simulink model "PM_fnc100_TestHarness_backup"  (R2022a)
settings: Solver=VariableStepAuto  StartTime=0.0  StopTime=10.0  RelTol=1e-3
values from neighbouring files (symbols this model uses):
  rate_ms = 10    [PM_fnc1000_tc01_iter01_testsignal_builder.m]    (also in PM_fnc21_tc01_iter01_testsignal_builder.m; PM_fnc22_tc01_iter01_testsignal_builder.m)
undefined symbols (not defined in the file or in its folder): cal_abs_ampslimit_hyst_A, cal_abs_ampslimit_thresh_A, cal_cell_heat2cool_factor, cal_Dchg_10sPL_expiry_dur_thresh_ms, cal_Dchg_50sPL_expiry_dur_thresh_ms, cal_Regen_10sPL_expiry_dur_thresh_ms, cal_Regen_50sPL_expiry_dur_thresh_ms, cal_table_cell_soc_percent, cal_table_cell_temp_degC
settings Model: Creator=306427  LastModifiedBy=306427

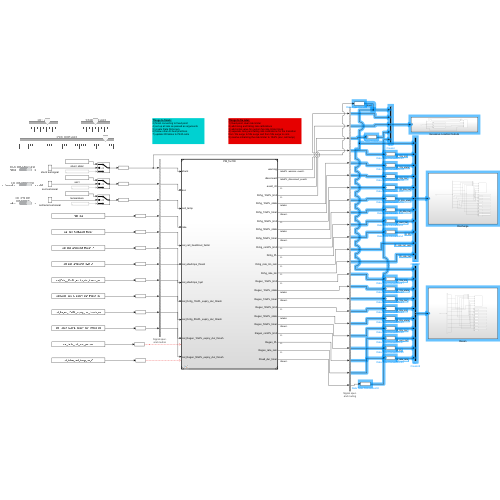
[thumbnail: Simulink's stored preview of the top-level diagram]
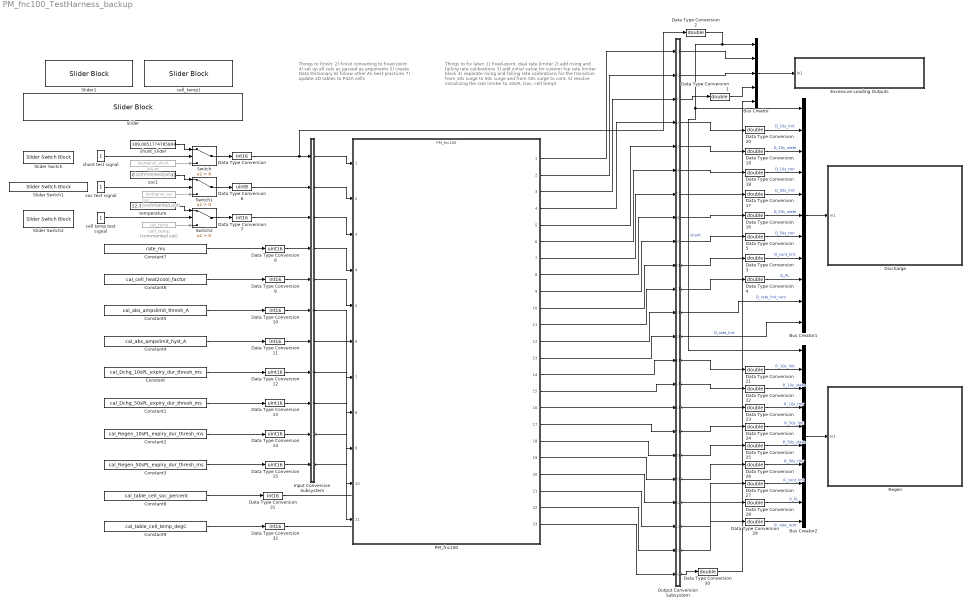
== system PM_fnc100_TestHarness_backup ==
  note: Things to finish:
      | 2) finish converting to fixed point
      | 4) set up all cals as passed as arguments
      | 5) create Data Dictionary
      | 6) follow other Ali best practices
      | 7) update 2D tables to P42A cells
  note: Things to fix later:
      | 1) fixed-point, dual rate limiter
      | 2) add rising and falling rate calibrations
      | 3) add initial value for custom fxp rate limiter block
      | 4) separate rising and falling rate calibrations for the transition from 10s surge to 50s surge and from 50s surge to cont.
      | 5) resolve initializing the rate limiter to 10sPL (soc, cell temp)
  Bus Creator : BusCreator  Inputs=5
  Bus Creator1 : BusCreator  Inputs=11
  Bus Creator2 : BusCreator  Inputs=10
  Constant : Constant  Value=cal_Dchg_10sPL_expiry_dur_thresh_ms
  Constant1 : Constant  Value=cal_Dchg_50sPL_expiry_dur_thresh_ms
  Constant2 : Constant  Value=cal_Regen_10sPL_expiry_dur_thresh_ms
  Constant3 : Constant  Value=cal_Regen_50sPL_expiry_dur_thresh_ms
  Constant4 : Constant  Value=cal_abs_ampslimit_hyst_A
  Constant5 : Constant  Value=cal_abs_ampslimit_thresh_A
  Constant6 : Constant  Value=cal_cell_heat2cool_factor
  Constant7 : Constant  Value=rate_ms
  Constant8 : Constant  Value=cal_table_cell_soc_percent
  Constant9 : Constant  Value=cal_table_cell_temp_degC
  Data Type Conversion{,7,9..11,31..32} (7 alike) : DataTypeConversion  OutDataTypeStr=int16  SaturateOnIntegerOverflow=off  RndMeth=Floor
  Data Type Conversion{1..5,16..30} (20 alike) : DataTypeConversion  OutDataTypeStr=double  SaturateOnIntegerOverflow=off  RndMeth=Floor
  Data Type Conversion{8,12..15} (5 alike) : DataTypeConversion  OutDataTypeStr=uint16  SaturateOnIntegerOverflow=off  RndMeth=Floor
  Data Type Conversion6 : DataTypeConversion  OutDataTypeStr=uint8  SaturateOnIntegerOverflow=off  RndMeth=Floor
  Discharge : Subsystem
  Excessive Loading Outputs : Subsystem
  Input Conversion Subsystem : Subsystem  Tag=__SLT_ICS__  Description=|
      | Signal spec.
      | and routing
      settings: AttributesFormatString=%<Description>
  Output Conversion Subsystem : Subsystem  Tag=__SLT_OCS__  Description=|
      | Signal spec.
      | and routing
      settings: AttributesFormatString=%<Description>
  PM_fnc100 : ModelReference  ModelNameDialog=PM_fnc100  SimulationMode=Normal  ModelReferenceVersion=1.79
  Regen : Subsystem
  Slider : SliderBlock  ScaleMin=-1700  ScaleMax=+500
  Slider Switch : SliderSwitchBlock
      settings: Values={{'from wksp', 'slider'}, [0 1]}
  Slider Switch1 : SliderSwitchBlock
      settings: Values={{'soc from wksp', 'soc slider'}, [0 1]}
  Slider Switch2 : SliderSwitchBlock
      settings: Values={{'from wksp', 'slider'}, [0 1]}
  Slider1 : SliderBlock
  Switch : Switch  Criteria=u2 > Threshold  SaturateOnIntegerOverflow=off  InputSameDT=off
  Switch1 : Switch  Criteria=u2 > Threshold  SaturateOnIntegerOverflow=off  InputSameDT=off
  Switch2 : Switch  Criteria=u2 > Threshold  SaturateOnIntegerOverflow=off  InputSameDT=off
  cell temp test signal : Constant
  cell_temp : FromWorkspace  Commented=on  VariableName=cell_temp  OutDataTypeStr=double  SampleTime=[0, 1]
  cell_temp1 : SliderBlock  ScaleMin=-20  ScaleMax=65
  shunt : FromWorkspace  Commented=on  VariableName=testsignal_shunt  OutDataTypeStr=double
  shunt test signal : Constant
  shunt_slider : Constant  Value=309.0651774785804  OutDataTypeStr=double
  soc : FromWorkspace  Commented=on  VariableName=testsignal_soc  OutDataTypeStr=double  SampleTime=[0, 1]
  soc test signal : Constant
  soc1 : Constant  Value=62.85016977928692  OutDataTypeStr=double
  temperature : Constant  Value=22.31058998302207  OutDataTypeStr=double
  wires:
  Data Type Conversion10/1 -> Input Conversion Subsystem/6(Inport_6)
  Input Conversion Subsystem/1(Outport_1) -> PM_fnc100/1
  Input Conversion Subsystem/3(Outport_3) -> PM_fnc100/3
  Data Type Conversion30/1 -> Bus Creator/5
  PM_fnc100/23 -> Output Conversion Subsystem/23(Inport_23)
  Bus Creator1/1 -> Discharge/1(In1)
  Output Conversion Subsystem/6(Outport_6) -> Data Type Conversion18/1
  Input Conversion Subsystem/7(Outport_7) -> PM_fnc100/7
  Data Type Conversion2/1 -> Bus Creator2/1, Bus Creator1/1, Bus Creator/1  "shunt"
  Input Conversion Subsystem/5(Outport_5) -> PM_fnc100/5
  Constant6/1 -> Data Type Conversion9/1
  Constant9/1 -> Data Type Conversion32/1
  Constant8/1 -> Data Type Conversion31/1
  PM_fnc100/12 -> Output Conversion Subsystem/12(Inport_12)
  Input Conversion Subsystem/11(Outport_11) -> PM_fnc100/11
  PM_fnc100/14 -> Output Conversion Subsystem/14(Inport_14)
  Data Type Conversion24/1 -> Bus Creator2/5  "R_50s_lmt"
  Output Conversion Subsystem/23(Outport_23) -> Data Type Conversion30/1
  Input Conversion Subsystem/8(Outport_8) -> PM_fnc100/8
  PM_fnc100/22 -> Output Conversion Subsystem/22(Inport_22)
  Constant/1 -> Data Type Conversion12/1
  Input Conversion Subsystem/2(Outport_2) -> PM_fnc100/2
  Input Conversion Subsystem/9(Outport_9) -> PM_fnc100/9
  Input Conversion Subsystem/6(Outport_6) -> PM_fnc100/6
  Data Type Conversion8/1 -> Input Conversion Subsystem/4(Inport_4)
  Output Conversion Subsystem/17(Outport_17) -> Data Type Conversion24/1
  soc/1 -> Switch1/3
  Switch2/1 -> Data Type Conversion7/1
  Data Type Conversion17/1 -> Bus Creator1/5  "D_50s_lmt"
  Data Type Conversion19/1 -> Bus Creator1/3  "D_10s_state"
  PM_fnc100/21 -> Output Conversion Subsystem/21(Inport_21)
  PM_fnc100/18 -> Output Conversion Subsystem/18(Inport_18)
  Output Conversion Subsystem/13(Outport_13) -> Bus Creator1/11  "D_rate_lmt"
  PM_fnc100/20 -> Output Conversion Subsystem/20(Inport_20)
  Input Conversion Subsystem/10(Outport_10) -> PM_fnc100/10
  soc test signal/1 -> Switch1/2
  Input Conversion Subsystem/4(Outport_4) -> PM_fnc100/4
  Data Type Conversion16/1 -> Bus Creator1/6  "D_50s_state"
  PM_fnc100/13 -> Output Conversion Subsystem/13(Inport_13)
  PM_fnc100/17 -> Output Conversion Subsystem/17(Inport_17)
  Constant2/1 -> Data Type Conversion14/1
  Data Type Conversion/1 -> Data Type Conversion2/1, Input Conversion Subsystem/1(Inport_1)
  Output Conversion Subsystem/14(Outport_14) -> Data Type Conversion21/1
  Output Conversion Subsystem/20(Outport_20) -> Data Type Conversion27/1
  PM_fnc100/16 -> Output Conversion Subsystem/16(Inport_16)
  PM_fnc100/10 -> Output Conversion Subsystem/10(Inport_10)
  PM_fnc100/11 -> Output Conversion Subsystem/11(Inport_11)
  PM_fnc100/15 -> Output Conversion Subsystem/15(Inport_15)
  shunt/1 -> Switch/3
  PM_fnc100/6 -> Output Conversion Subsystem/6(Inport_6)
  Data Type Conversion26/1 -> Bus Creator2/7  "R_50s_tmr"
  PM_fnc100/3 -> Output Conversion Subsystem/3(Inport_3)
  Data Type Conversion5/1 -> Bus Creator1/7  "D_50s_tmr"
  PM_fnc100/5 -> Output Conversion Subsystem/5(Inport_5)
  PM_fnc100/8 -> Output Conversion Subsystem/8(Inport_8)
  Data Type Conversion7/1 -> Input Conversion Subsystem/3(Inport_3)
  Data Type Conversion6/1 -> Input Conversion Subsystem/2(Inport_2)
  Data Type Conversion13/1 -> Input Conversion Subsystem/9(Inport_9)
  Data Type Conversion21/1 -> Bus Creator2/2  "R_10s_lmt"
  Constant7/1 -> Data Type Conversion8/1
  Data Type Conversion15/1 -> Input Conversion Subsystem/11(Inport_11)
  Data Type Conversion22/1 -> Bus Creator2/3  "R_10s_state"
  Data Type Conversion14/1 -> Input Conversion Subsystem/10(Inport_10)
  Data Type Conversion28/1 -> Bus Creator2/9  "R_PL"
  Data Type Conversion1/1 -> Bus Creator/4
  Data Type Conversion27/1 -> Bus Creator2/8  "R_cont_lmt"
  Bus Creator2/1 -> Regen/1(In1)
  PM_fnc100/19 -> Output Conversion Subsystem/19(Inport_19)
  Output Conversion Subsystem/21(Outport_21) -> Data Type Conversion28/1
  Output Conversion Subsystem/5(Outport_5) -> Data Type Conversion19/1
  soc1/1 -> Switch1/1
  Output Conversion Subsystem/19(Outport_19) -> Data Type Conversion26/1
  Output Conversion Subsystem/10(Outport_10) -> Data Type Conversion3/1
  Data Type Conversion3/1 -> Bus Creator1/8  "D_cont_lmt"
  Output Conversion Subsystem/12(Outport_12) -> Bus Creator1/10  "D_rate_lmt_rem"
  Output Conversion Subsystem/16(Outport_16) -> Data Type Conversion23/1
  Switch1/1 -> Data Type Conversion6/1
  PM_fnc100/7 -> Output Conversion Subsystem/7(Inport_7)
  Constant5/1 -> Data Type Conversion10/1
  temperature/1 -> Switch2/1
  shunt test signal/1 -> Switch/2
  Output Conversion Subsystem/18(Outport_18) -> Data Type Conversion25/1
  cell temp test signal/1 -> Switch2/2
  PM_fnc100/9 -> Output Conversion Subsystem/9(Inport_9)
  shunt_slider/1 -> Switch/1
  Bus Creator/1 -> Excessive Loading Outputs/1(In1)
  Data Type Conversion23/1 -> Bus Creator2/4  "R_10s_tmr"
  Output Conversion Subsystem/8(Outport_8) -> Data Type Conversion16/1
  Data Type Conversion9/1 -> Input Conversion Subsystem/5(Inport_5)
  Output Conversion Subsystem/22(Outport_22) -> Data Type Conversion29/1
  Output Conversion Subsystem/7(Outport_7) -> Data Type Conversion17/1
  Output Conversion Subsystem/3(Outport_3) -> Data Type Conversion1/1
  Data Type Conversion20/1 -> Bus Creator1/2  "D_10s_lmt"
  Constant4/1 -> Data Type Conversion11/1
  Data Type Conversion25/1 -> Bus Creator2/6  "R_50s_state"
  Output Conversion Subsystem/1(Outport_1) -> Bus Creator/2
  PM_fnc100/4 -> Output Conversion Subsystem/4(Inport_4)
  Constant3/1 -> Data Type Conversion15/1
  Switch/1 -> Data Type Conversion/1
  Output Conversion Subsystem/15(Outport_15) -> Data Type Conversion22/1
  Data Type Conversion11/1 -> Input Conversion Subsystem/7(Inport_7)
  Data Type Conversion18/1 -> Bus Creator1/4  "D_10s_tmr"
  Constant1/1 -> Data Type Conversion13/1
  Output Conversion Subsystem/2(Outport_2) -> Bus Creator/3
  Data Type Conversion4/1 -> Bus Creator1/9  "D_PL"
  cell_temp/1 -> Switch2/3
  PM_fnc100/2 -> Output Conversion Subsystem/2(Inport_2)
  Output Conversion Subsystem/4(Outport_4) -> Data Type Conversion20/1
  Data Type Conversion31/1 -> ?
  Data Type Conversion12/1 -> Input Conversion Subsystem/8(Inport_8)
  Data Type Conversion29/1 -> Bus Creator2/10  "R_rate_rem"
  Data Type Conversion32/1 -> ?
  PM_fnc100/1 -> Output Conversion Subsystem/1(Inport_1)
  Output Conversion Subsystem/9(Outport_9) -> Data Type Conversion5/1
  Output Conversion Subsystem/11(Outport_11) -> Data Type Conversion4/1

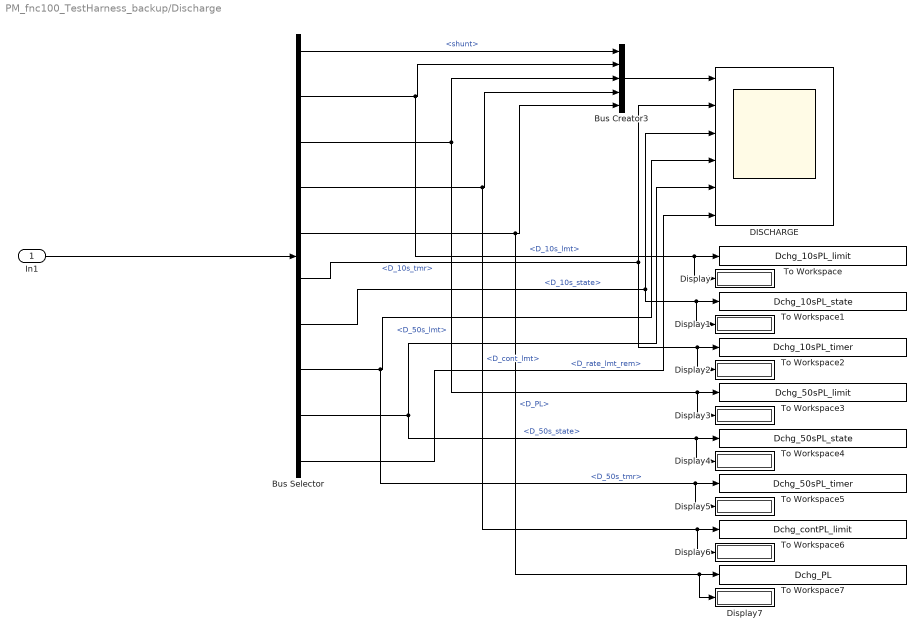
== system PM_fnc100_TestHarness_backup/Discharge ==
  In1 : Inport
  Bus Creator3 : BusCreator  Inputs=5
  Bus Selector : BusSelector  OutputSignals=shunt,D_10s_lmt,D_50s_lmt,D_cont_lmt,D_PL,D_10s_tmr,D_10s_state,D_50s_tmr,D_50s_state,D_rate_lmt_rem
  DISCHARGE : Scope  NumInputPorts=6
  Display{,1..7} (8 alike) : Display
  To Workspace : ToWorkspace  VariableName=Dchg_10sPL_limit  SampleTime=-1
      settings: Save2DSignal=2-D array (concatenate along first dimension)
  To Workspace1 : ToWorkspace  VariableName=Dchg_10sPL_state  SampleTime=-1
      settings: Save2DSignal=2-D array (concatenate along first dimension)
  To Workspace2 : ToWorkspace  VariableName=Dchg_10sPL_timer  SampleTime=-1
      settings: Save2DSignal=2-D array (concatenate along first dimension)
  To Workspace3 : ToWorkspace  VariableName=Dchg_50sPL_limit  SampleTime=-1
      settings: Save2DSignal=2-D array (concatenate along first dimension)
  To Workspace4 : ToWorkspace  VariableName=Dchg_50sPL_state  SampleTime=-1
      settings: Save2DSignal=2-D array (concatenate along first dimension)
  To Workspace5 : ToWorkspace  VariableName=Dchg_50sPL_timer  SampleTime=-1
      settings: Save2DSignal=2-D array (concatenate along first dimension)
  To Workspace6 : ToWorkspace  VariableName=Dchg_contPL_limit  SampleTime=-1
      settings: Save2DSignal=2-D array (concatenate along first dimension)
  To Workspace7 : ToWorkspace  VariableName=Dchg_PL  SampleTime=-1
      settings: Save2DSignal=2-D array (concatenate along first dimension)
  wires:
  Bus Selector/5 -> To Workspace7/1, Display7/1, Bus Creator3/5  "<D_PL>"
  Bus Selector/9 -> DISCHARGE/5, To Workspace4/1, Display4/1  "<D_50s_state>"
  Bus Selector/2 -> To Workspace/1, Display/1, Bus Creator3/2  "<D_10s_lmt>"
  Bus Selector/4 -> To Workspace6/1, Display6/1, Bus Creator3/4  "<D_cont_lmt>"
  Bus Selector/7 -> DISCHARGE/3, To Workspace1/1, Display1/1  "<D_10s_state>"
  Bus Selector/6 -> To Workspace2/1, Display2/1, DISCHARGE/2  "<D_10s_tmr>"
  Bus Selector/10 -> DISCHARGE/6  "<D_rate_lmt_rem>"
  Bus Selector/8 -> To Workspace5/1, Display5/1, DISCHARGE/4  "<D_50s_tmr>"
  Bus Selector/3 -> To Workspace3/1, Display3/1, Bus Creator3/3  "<D_50s_lmt>"
  Bus Selector/1 -> Bus Creator3/1  "<shunt>"
  Bus Creator3/1 -> DISCHARGE/1
  In1/1 -> Bus Selector/1

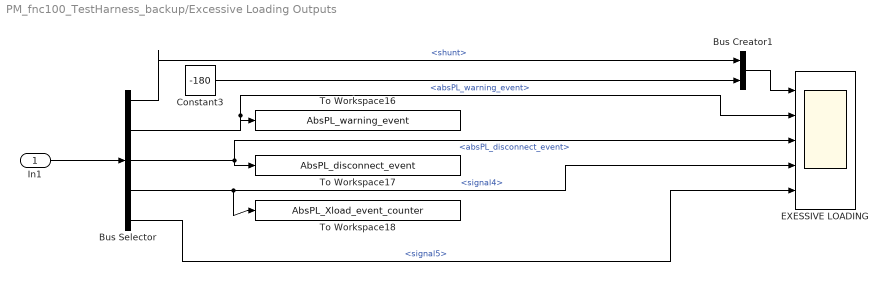
== system PM_fnc100_TestHarness_backup/Excessive Loading Outputs ==
  In1 : Inport
  Bus Creator1 : BusCreator  Inputs=2
  Bus Selector : BusSelector  OutputSignals=shunt,absPL_warning_event,absPL_disconnect_event,signal4,signal5
  Constant3 : Constant  Value=-180  OutDataTypeStr=double
  EXESSIVE LOADING : Scope  NumInputPorts=5
  To Workspace16 : ToWorkspace  VariableName=AbsPL_warning_event  SampleTime=-1
      settings: Save2DSignal=2-D array (concatenate along first dimension)
  To Workspace17 : ToWorkspace  VariableName=AbsPL_disconnect_event  SampleTime=-1
      settings: Save2DSignal=2-D array (concatenate along first dimension)
  To Workspace18 : ToWorkspace  VariableName=AbsPL_Xload_event_counter  SampleTime=-1
      settings: Save2DSignal=2-D array (concatenate along first dimension)
  wires:
  In1/1 -> Bus Selector/1
  Bus Selector/2 -> EXESSIVE LOADING/2, To Workspace16/1  "<absPL_warning_event>"
  Constant3/1 -> Bus Creator1/2
  Bus Selector/3 -> To Workspace17/1, EXESSIVE LOADING/3  "<absPL_disconnect_event>"
  Bus Creator1/1 -> EXESSIVE LOADING/1
  Bus Selector/1 -> Bus Creator1/1  "<shunt>"
  Bus Selector/4 -> To Workspace18/1, EXESSIVE LOADING/4  "<signal4>"
  Bus Selector/5 -> EXESSIVE LOADING/5  "<signal5>"

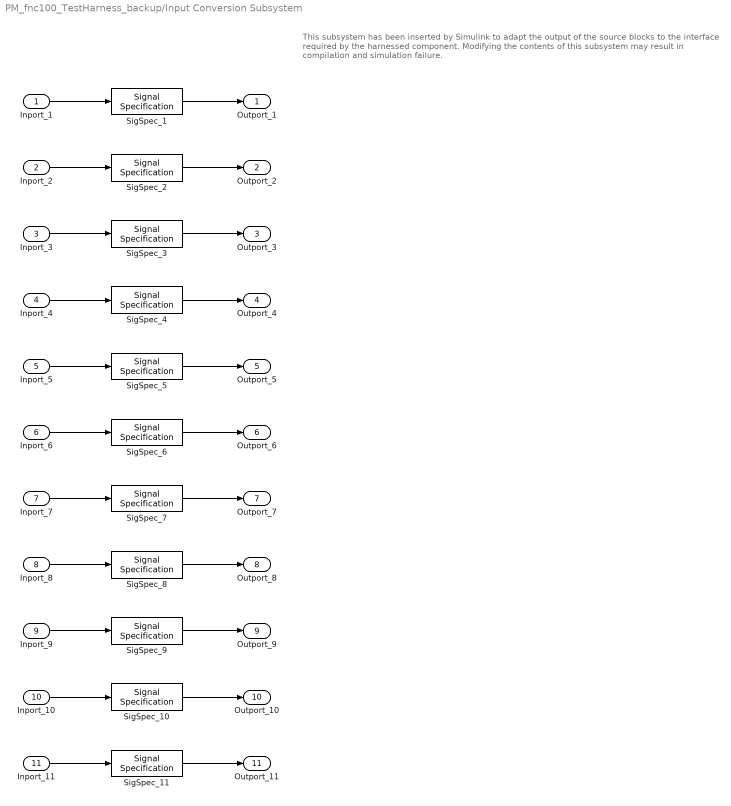
== system PM_fnc100_TestHarness_backup/Input Conversion Subsystem ==
  note: This subsystem has been inserted by Simulink to adapt the output of the source blocks to the interface required by the harnessed component.
      |  Modifying the contents of this subsystem may result in compilation and simulation failure.
  Inport_1 : Inport
  Inport_2 : Inport  Port=2
  Inport_3 : Inport  Port=3
  Inport_4 : Inport  Port=4
  Inport_5 : Inport  Port=5
  Inport_6 : Inport  Port=6
  Inport_7 : Inport  Port=7
  Inport_8 : Inport  Port=8
  Inport_9 : Inport  Port=9
  Inport_10 : Inport  Port=10
  Inport_11 : Inport  Port=11
  SigSpec_1 : SignalSpecification  OutDataTypeStr=int16  Unit=A  Dimensions=[1]  SampleTime=0.01
  SigSpec_{4,8..11} (5 alike) : SignalSpecification  OutDataTypeStr=uint16  Unit=msec  Dimensions=[1]  SampleTime=0.01
  SigSpec_2 : SignalSpecification  OutDataTypeStr=uint8  Unit=%  Dimensions=[1]  SampleTime=0.01
  SigSpec_3 : SignalSpecification  OutDataTypeStr=int16  Unit=°C  Dimensions=[1]  SampleTime=0.01
  SigSpec_5 : SignalSpecification  OutDataTypeStr=int16  Dimensions=[1]  SampleTime=0.01
  SigSpec_6 : SignalSpecification  OutDataTypeStr=int16  Unit=A  Dimensions=[1]  SampleTime=0.01
  SigSpec_7 : SignalSpecification  OutDataTypeStr=int16  Unit=A  Dimensions=[1]  SampleTime=0.01
  Outport_1 : Outport
  Outport_2 : Outport  Port=2
  Outport_3 : Outport  Port=3
  Outport_4 : Outport  Port=4
  Outport_5 : Outport  Port=5
  Outport_6 : Outport  Port=6
  Outport_7 : Outport  Port=7
  Outport_8 : Outport  Port=8
  Outport_9 : Outport  Port=9
  Outport_10 : Outport  Port=10
  Outport_11 : Outport  Port=11
  wires:
  SigSpec_1/1 -> Outport_1/1
  Inport_1/1 -> SigSpec_1/1
  SigSpec_2/1 -> Outport_2/1
  Inport_2/1 -> SigSpec_2/1
  SigSpec_3/1 -> Outport_3/1
  Inport_3/1 -> SigSpec_3/1
  SigSpec_4/1 -> Outport_4/1
  Inport_4/1 -> SigSpec_4/1
  SigSpec_5/1 -> Outport_5/1
  Inport_5/1 -> SigSpec_5/1
  SigSpec_6/1 -> Outport_6/1
  Inport_6/1 -> SigSpec_6/1
  SigSpec_7/1 -> Outport_7/1
  Inport_7/1 -> SigSpec_7/1
  SigSpec_8/1 -> Outport_8/1
  Inport_8/1 -> SigSpec_8/1
  SigSpec_9/1 -> Outport_9/1
  Inport_9/1 -> SigSpec_9/1
  SigSpec_10/1 -> Outport_10/1
  Inport_10/1 -> SigSpec_10/1
  SigSpec_11/1 -> Outport_11/1
  Inport_11/1 -> SigSpec_11/1

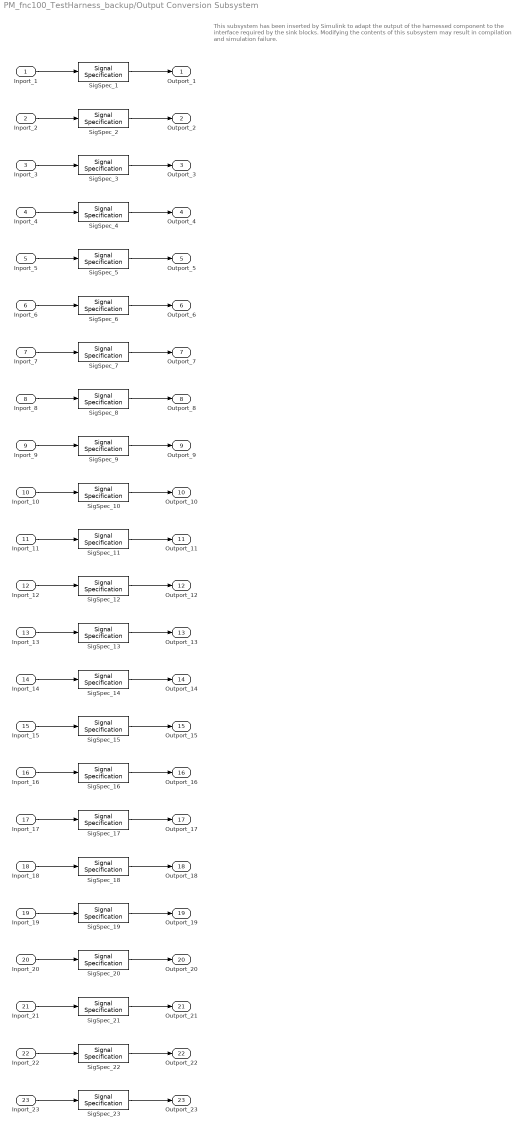
== system PM_fnc100_TestHarness_backup/Output Conversion Subsystem ==
  note: This subsystem has been inserted by Simulink to adapt the output of the harnessed component to the interface required by the sink blocks.
      |  Modifying the contents of this subsystem may result in compilation and simulation failure.
  Inport_1 : Inport
  Inport_2 : Inport  Port=2
  Inport_3 : Inport  Port=3
  Inport_4 : Inport  Port=4
  Inport_5 : Inport  Port=5
  Inport_6 : Inport  Port=6
  Inport_7 : Inport  Port=7
  Inport_8 : Inport  Port=8
  Inport_9 : Inport  Port=9
  Inport_10 : Inport  Port=10
  Inport_11 : Inport  Port=11
  Inport_12 : Inport  Port=12
  Inport_13 : Inport  Port=13
  Inport_14 : Inport  Port=14
  Inport_15 : Inport  Port=15
  Inport_16 : Inport  Port=16
  Inport_17 : Inport  Port=17
  Inport_18 : Inport  Port=18
  Inport_19 : Inport  Port=19
  Inport_20 : Inport  Port=20
  Inport_21 : Inport  Port=21
  Inport_22 : Inport  Port=22
  Inport_23 : Inport  Port=23
  SigSpec_1 : SignalSpecification  OutDataTypeStr=boolean  Dimensions=[1]  SampleTime=0.01
  SigSpec_{4,7,10..14,17,20..21} (10 alike) : SignalSpecification  OutDataTypeStr=int16  Unit=A  Dimensions=[1]  SampleTime=0.01
  SigSpec_{5,8,15,18} (4 alike) : SignalSpecification  OutDataTypeStr=uint8  Dimensions=[1]  SampleTime=0.01
  SigSpec_{6,9,16,19} (4 alike) : SignalSpecification  OutDataTypeStr=uint16  Unit=msec  Dimensions=[1]  SampleTime=0.01
  SigSpec_2 : SignalSpecification  OutDataTypeStr=boolean  Dimensions=[1]  SampleTime=0.01
  SigSpec_22 : SignalSpecification  OutDataTypeStr=int32  Unit=A  Dimensions=[1]  SampleTime=0.01
  SigSpec_23 : SignalSpecification  OutDataTypeStr=uint16  Dimensions=[1]  SampleTime=0.01
  SigSpec_3 : SignalSpecification  OutDataTypeStr=uint16  Dimensions=[1]  SampleTime=0.01
  Outport_1 : Outport
  Outport_2 : Outport  Port=2
  Outport_3 : Outport  Port=3
  Outport_4 : Outport  Port=4
  Outport_5 : Outport  Port=5
  Outport_6 : Outport  Port=6
  Outport_7 : Outport  Port=7
  Outport_8 : Outport  Port=8
  Outport_9 : Outport  Port=9
  Outport_10 : Outport  Port=10
  Outport_11 : Outport  Port=11
  Outport_12 : Outport  Port=12
  Outport_13 : Outport  Port=13
  Outport_14 : Outport  Port=14
  Outport_15 : Outport  Port=15
  Outport_16 : Outport  Port=16
  Outport_17 : Outport  Port=17
  Outport_18 : Outport  Port=18
  Outport_19 : Outport  Port=19
  Outport_20 : Outport  Port=20
  Outport_21 : Outport  Port=21
  Outport_22 : Outport  Port=22
  Outport_23 : Outport  Port=23
  wires:
  Inport_1/1 -> SigSpec_1/1
  SigSpec_1/1 -> Outport_1/1
  Inport_2/1 -> SigSpec_2/1
  SigSpec_2/1 -> Outport_2/1
  Inport_3/1 -> SigSpec_3/1
  SigSpec_3/1 -> Outport_3/1
  Inport_4/1 -> SigSpec_4/1
  SigSpec_4/1 -> Outport_4/1
  Inport_5/1 -> SigSpec_5/1
  SigSpec_5/1 -> Outport_5/1
  Inport_6/1 -> SigSpec_6/1
  SigSpec_6/1 -> Outport_6/1
  Inport_7/1 -> SigSpec_7/1
  SigSpec_7/1 -> Outport_7/1
  Inport_8/1 -> SigSpec_8/1
  SigSpec_8/1 -> Outport_8/1
  Inport_9/1 -> SigSpec_9/1
  SigSpec_9/1 -> Outport_9/1
  Inport_10/1 -> SigSpec_10/1
  SigSpec_10/1 -> Outport_10/1
  Inport_11/1 -> SigSpec_11/1
  SigSpec_11/1 -> Outport_11/1
  Inport_12/1 -> SigSpec_12/1
  SigSpec_12/1 -> Outport_12/1
  Inport_13/1 -> SigSpec_13/1
  SigSpec_13/1 -> Outport_13/1
  Inport_14/1 -> SigSpec_14/1
  SigSpec_14/1 -> Outport_14/1
  Inport_15/1 -> SigSpec_15/1
  SigSpec_15/1 -> Outport_15/1
  Inport_16/1 -> SigSpec_16/1
  SigSpec_16/1 -> Outport_16/1
  Inport_17/1 -> SigSpec_17/1
  SigSpec_17/1 -> Outport_17/1
  Inport_18/1 -> SigSpec_18/1
  SigSpec_18/1 -> Outport_18/1
  Inport_19/1 -> SigSpec_19/1
  SigSpec_19/1 -> Outport_19/1
  Inport_20/1 -> SigSpec_20/1
  SigSpec_20/1 -> Outport_20/1
  Inport_21/1 -> SigSpec_21/1
  SigSpec_21/1 -> Outport_21/1
  Inport_22/1 -> SigSpec_22/1
  SigSpec_22/1 -> Outport_22/1
  Inport_23/1 -> SigSpec_23/1
  SigSpec_23/1 -> Outport_23/1

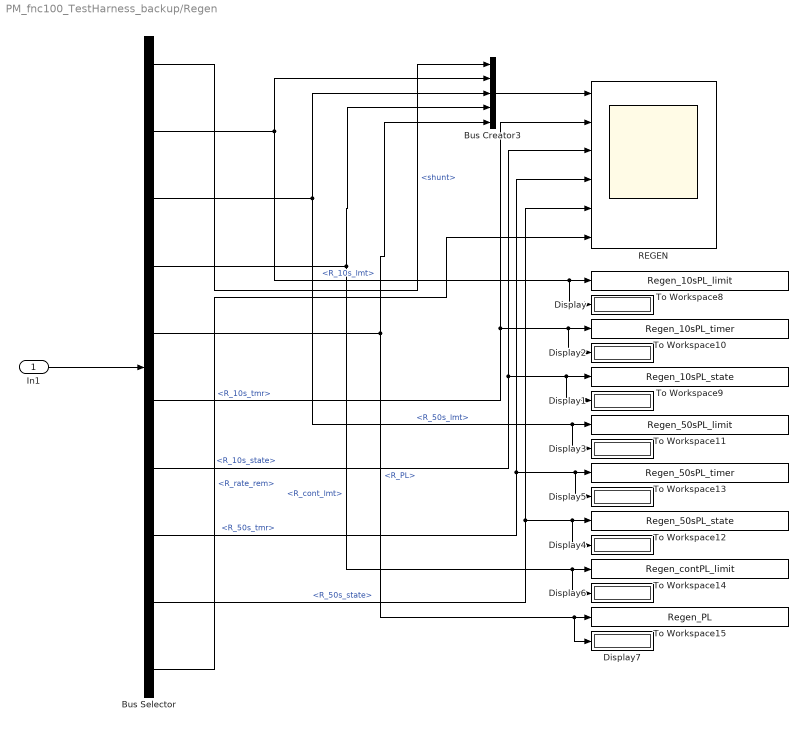
== system PM_fnc100_TestHarness_backup/Regen ==
  In1 : Inport
  Bus Creator3 : BusCreator  Inputs=5
  Bus Selector : BusSelector  OutputSignals=shunt,R_10s_lmt,R_50s_lmt,R_cont_lmt,R_PL,R_10s_tmr,R_10s_state,R_50s_tmr,R_50s_state,R_rate_rem
  Display{,1..7} (8 alike) : Display
  REGEN : Scope  NumInputPorts=6
  To Workspace10 : ToWorkspace  VariableName=Regen_10sPL_timer  SampleTime=-1
      settings: Save2DSignal=2-D array (concatenate along first dimension)
  To Workspace11 : ToWorkspace  VariableName=Regen_50sPL_limit  SampleTime=-1
      settings: Save2DSignal=2-D array (concatenate along first dimension)
  To Workspace12 : ToWorkspace  VariableName=Regen_50sPL_state  SampleTime=-1
      settings: Save2DSignal=2-D array (concatenate along first dimension)
  To Workspace13 : ToWorkspace  VariableName=Regen_50sPL_timer  SampleTime=-1
      settings: Save2DSignal=2-D array (concatenate along first dimension)
  To Workspace14 : ToWorkspace  VariableName=Regen_contPL_limit  SampleTime=-1
      settings: Save2DSignal=2-D array (concatenate along first dimension)
  To Workspace15 : ToWorkspace  VariableName=Regen_PL  SampleTime=-1
      settings: Save2DSignal=2-D array (concatenate along first dimension)
  To Workspace8 : ToWorkspace  VariableName=Regen_10sPL_limit  SampleTime=-1
      settings: Save2DSignal=2-D array (concatenate along first dimension)
  To Workspace9 : ToWorkspace  VariableName=Regen_10sPL_state  SampleTime=-1
      settings: Save2DSignal=2-D array (concatenate along first dimension)
  wires:
  Bus Selector/5 -> To Workspace15/1, Display7/1, Bus Creator3/5  "<R_PL>"
  Bus Selector/2 -> To Workspace8/1, Display/1, Bus Creator3/2  "<R_10s_lmt>"
  Bus Selector/4 -> To Workspace14/1, Display6/1, Bus Creator3/4  "<R_cont_lmt>"
  Bus Selector/3 -> To Workspace11/1, Display3/1, Bus Creator3/3  "<R_50s_lmt>"
  Bus Selector/1 -> Bus Creator3/1  "<shunt>"
  Bus Creator3/1 -> REGEN/1
  In1/1 -> Bus Selector/1
  Bus Selector/10 -> REGEN/6  "<R_rate_rem>"
  Bus Selector/6 -> REGEN/2, Display2/1, To Workspace10/1  "<R_10s_tmr>"
  Bus Selector/7 -> REGEN/3, Display1/1, To Workspace9/1  "<R_10s_state>"
  Bus Selector/8 -> REGEN/4, Display5/1, To Workspace13/1  "<R_50s_tmr>"
  Bus Selector/9 -> REGEN/5, Display4/1, To Workspace12/1  "<R_50s_state>"
